simulink model "WormAndGearConstraint0x5B10x5D"  (R2024a)
settings: Solver=ode45  StartTime=0.0  StopTime=20  MaxStep=0.01  RelTol=1e-3
PreLoadFcn:
  | addpath(fullfile('WormAndGearConstraintSupport','Data'));
  | addpath(fullfile('WormAndGearConstraintSupport','Scripts'));
model workspace: external: MATLAB File WormAndGearConstraintParameters.m (data not in the file)
undefined symbols (not defined in the file): driveconn, frame, framemount, slewdrive, solarpanel, support, X, Y, Z
libraries: sm_lib x393, nesl_utility x10, fl_lib x4, SignalEditorBlockLib x2, fl_ps_legacy_lib x1
(part 2 of 11)

== system WormAndGearConstraint0x5B10x5D/Solar Array/Solar Tracker1/Slew Drive ==
  Housing : Subsystem
      mask Display:
      | image(fullfile('WormAndGearConstraintSupport','Images','SlewDriveHousing.png'));
      | port_label('lconn',1,'S');
      | port_label('rconn',1,'B');
  Housing xForm : sm_lib/Frames and Transforms/Rigid Transform  RotationMethod=AlignedAxes  FollAlignAxisA=+X  BaseAlignAxisA=-Y  FollAlignAxisB=+Z  BaseAlignAxisB=+Z  RotationStandardAxis=+Z  RotationAngle=0.0  RotationAngleUnits=deg  RotationArbitraryAxis=[0 0 1]  RotationSequenceAxes=FollowerAxes  RotationSequence=XYX  RotationSequenceAngles=[0 0 0]  RotationSequenceAnglesUnits=deg  RotationMatrix=[1 0 0; 0 1 0; 0 0 1]  Quaternion=[1 0 0 0]  TranslationMethod=StandardAxis  TranslationCartesianOffset=[0 0 0]  TranslationCartesianOffsetUnits=m  TranslationStandardAxis=+Y  TranslationStandardOffset=housingOffset  TranslationStandardOffsetUnits=m  TranslationROffset=0  TranslationROffsetUnits=m  TranslationThetaOffset=0  TranslationThetaOffsetUnits=deg  TranslationZOffset=0  TranslationZOffsetUnits=m
  Root Frame : sm_lib/Frames and Transforms/Reference Frame
  Worm and Gear Assembly : Subsystem
      mask Display:
      | image(fullfile('WormAndGearConstraintSupport','Images','SlewDriveWormAndGear.png'));
      | port_label('lconn',1,'R');
      | port_label('lconn',2,'qGear');
      | port_label('rconn',1,'T');
      | port_label('rconn',2,'wWorm');
      | port_label('rconn',3,'tWorm');
  B : PMIOPort  Side=Left
  T : PMIOPort  Port=2  Side=Right
  qGear : PMIOPort  Port=3  Side=Left
  wWorm : PMIOPort  Port=4  Side=Right
  tWorm : PMIOPort  Port=5  Side=Right
  connections:
  qGear/RConn1 -- Worm and Gear Assembly/LConn2
  tWorm/RConn1 -- Worm and Gear Assembly/RConn3
  Worm and Gear Assembly/RConn2 -- wWorm/RConn1
  T/RConn1 -- Worm and Gear Assembly/RConn1
  Housing xForm/LConn1 -- Worm and Gear Assembly/LConn1 -- Root Frame/RConn1
  B/RConn1 -- Housing/RConn1
  Housing/LConn1 -- Housing xForm/RConn1

== system WormAndGearConstraint0x5B10x5D/Solar Array/Solar Tracker1/Solar Panel Assembly ==
  Frame : Subsystem  AncestorBlock=WormAndGearConstraintLibrary/Frame  mask(Frame){width=frame.width, height=frame.height, depth=frame.depth, beamWidth=frame.beamWidth, beamThickness=frame.beamThickness, frameWidth=frame.frameWidth, frameThickness=frame.frameThickness, rho=frame.density, beamColor=frame.beamColor, frameColor=frame.frameColor}
      mask prompts: width "Width (m)"; height "Height (m)"; depth "Depth (m)"; beamWidth "Beam Width (m)"; beamThickness "Beam Thickness (m)"; frameWidth "Frame Width (m)"; frameThickness "Frame Thickness (m)"; rho "Density (kg/m^3)"; beamColor "Beam Color [r g b]"; frameColor "Frame Color [r g b]"
      mask help:
      | This block models the mounting frame of the solar tracker.
      |
      | Port B corresponds to the center of the base face of the horizontal beam. Port T corresponds to the center of the top face of the horizontal beam.
      mask init:
      | horizBeamLength = width - 2*frameWidth;
      | vertBeamLength = height - 2*frameWidth;
      | 
      | vertBeam1_offset = [-0.5*vertBeamLength 0 -(1/3)*horizBeamLength];
      | vertBeam2_offset = [-0.5*vertBeamLength 0 -(2/3)*horizBeamLength];
      | 
      | baseOffset = [0 -0.5*depth 0.5*horizBeamLength];
      | topOffset  = [0  0.5*depth 0.5*horizBeamLength];
      | 
      | leftFrameOffset  = [-0.5*height 0 -0.5*frameWidth];
      | rightFrameOffset = [-0.5*height 0  0.5*frameWidth];
      | 
      | nearFarFrameOffset = 0.5*height-0.5*frameWidth;
      settings: LibrarySourceBlock=sm_solar_tracker_lib/Frame
      mask DialogControl Tab1 Prompt: Dimensions
      mask DialogControl Tab2 Prompt: Material Properties
      mask Display:
      | image(fullfile('WormAndGearConstraintSupport','Images','Frame.png'));
      | port_label('lconn',1,'B');
      | port_label('rconn',1,'T');
  Frame Mount : Subsystem  AncestorBlock=WormAndGearConstraintLibrary/Frame Mount  mask(Frame Mount){bracketWidth=framemount.bracketWidthHeight, bracketThickness=framemount.bracketThickness, bracketOffset=framemount.bracketOffset, holeRadius=framemount.holeRadius, holeOffset=framemount.holeOffset, baseThickness=framemount.baseThickness, rho=framemount.density, mountColor=framemount.mountColor, pinColor=framemount.pinColor}
      mask prompts: bracketWidth "Bracket Width and Height (m)"; bracketThickness "Bracket Thickness (m)"; bracketOffset "Bracket Offset (m)"; holeRadius "Hole Radius (m)"; holeOffset "Hole Offset (m)"; baseThickness "Base Thickness (m)"; rho "Density (kg/m^3)"; mountColor "Mount Color [r g b]"; pinColor "Pin Color [r g b]"
      mask help:
      | This block models the mount for the frame of the solar tracker.
      |
      | Port B corresponds to the center of the base plate. Port H corresponds to the center point of the pin that passes through the holes of the bracket.
      mask init:
      | baseAngle = atan(bracketWidth / (bracketOffset + bracketThickness));
      | baseRadius = 0.5*bracketWidth / sin(baseAngle);
      | pinLength = bracketOffset + bracketThickness;
      settings: LibrarySourceBlock=sm_solar_tracker_lib/Frame Mount
      mask DialogControl Tab1 Prompt: Dimensions
      mask DialogControl Tab2 Prompt: Material Properties
      mask Display:
      | image(fullfile('WormAndGearConstraintSupport','Images','FrameMount.png'));
      | port_label('lconn',1,'B');
      | port_label('rconn',1,'H');
  Solar Panel : Subsystem  AncestorBlock=WormAndGearConstraintLibrary/Solar Panel  mask(Solar Panel){width=solarpanel.width, height=solarpanel.height, frameWidth=solarpanel.frameWidth, frameDepth=solarpanel.frameDepth, cellsRho=solarpanel.cellDensity, frameRho=solarpanel.frameDensity, cellsColor=solarpanel.cellColor, frameColor=solarpanel.frameColor}
      mask prompts: width "Width (m)"; height "Height (m)"; frameWidth "Frame Width (m)"; frameDepth "Frame Depth (m)"; cellsRho "Cell Density (kg/m^3)"; frameRho "Frame Density (kg/m^3)"; cellsColor "Cell Color [r g b]"; frameColor "Frame Color [r g b]"
      mask help:
      | This block models the solar panel of the solar tracker.
      |
      | Port B corresponds to the center of the base face.
      mask init:
      | % Solar cells
      | cellsDim = ...
      |   [width-2*frameWidth, height-2*frameWidth, 0.25*frameDepth];
      | 
      | % Frame base and edges
      | frameBaseDim = [width height 0.25*frameDepth];
      | frameVertEdgeDim = [frameWidth height 0.75*frameDepth];
      | frameHorizEdgeDim = [width-2*frameWidth frameWidth 0.75*frameDepth];
      | 
      | % Horizontal dividers
      | frameMajorHorizDim = frameHorizEdgeDim;
      | frameMinorHorizDim = ...
      |   [width-2*frameWidth 0.5*frameWidth 0.25*frameDepth];
      | 
      | frameMinorHorizSpacing = (1/12)*(height-frameWidth);
      | frameMinorHorizOffsetZ = -0.25*frameDepth;
      | 
      | frameMinorHoriz1_offset  = ...
      |   [0  5*frameMinorHorizSpacing frameMinorHorizOffsetZ];
      | frameMinorHoriz2_offset  = ...
      |   [0  4*frameMinorHorizSpacing frameMinorHorizOffsetZ];
      | frameMinorHoriz3_offset  = ...
      |   [0  3*frameMinorHorizSpacing frameMinorHorizOffsetZ];
      | frameMinorHoriz4_offset  = ...
      |   [0  2*frameMinorHorizSpacing frameMinorHorizOffsetZ];
      | frameMinorHoriz5_offset  = ...
      |   [0  1*frameMinorHorizSpacing frameMinorHorizOffsetZ];
      | frameMinorHoriz6_offset  = ...
      |   [0 -1*frameMinorHorizSpacing frameMinorHorizOffsetZ];
      | frameMinorHoriz7_offset  = ...
      |   [0 -2*frameMinorHorizSpacing frameMinorHorizOffsetZ];
      | frameMinorHoriz8_offset  = ...
      |   [0 -3*frameMinorHorizSpacing frameMinorHorizOffsetZ];
      | frameMinorHoriz9_offset  = ...
      |   [0 -4*frameMinorHorizSpacing frameMinorHorizOffsetZ];
      | frameMinorHoriz10_offset = ...
      |   [0 -5*frameMinorHorizSpacing frameMinorHorizOffsetZ];
      | 
      | % Vertical dividers
      | frameMajorVertDim = ...
      |   [frameWidth height-2*frameWidth 0.5*frameDepth];
      | frameMinorVertDim = ...
      |   [0.25*frameWidth height-2*frameWidth 0.125*frameDepth];
      | 
      | frameMajorVertOffset = (1/6)*width;
      | frameMinorVertSpacing = (1/18)*(width-frameWidth);
      | frameMinorVertOffsetZ = -(0.5*frameDepth-frameMinorVertDim(3));
      | 
      | frameMinorVert1_offset = ...
      |   [-7*frameMinorVertSpacing 0 frameMinorVertOffsetZ];
      | frameMinorVert2_offset = ...
      |   [-5*frameMinorVertSpacing 0 frameMinorVertOffsetZ];
      | frameMinorVert3_offset = ...
      |   [-1*frameMinorVertSpacing 0 frameMinorVertOffsetZ];
      | frameMinorVert4_offset = ...
      |   [ 1*frameMinorVertSpacing 0 frameMinorVertOffsetZ];
      | frameMinorVert5_offset = ...
      |   [ 5*frameMinorVertSpacing 0 frameMinorVertOffsetZ];
      | frameMinorVert6_offset = ...
      |   [ 7*frameMinorVertSpacing 0 frameMinorVertOffsetZ];
      settings: LibrarySourceBlock=sm_solar_tracker_lib/Solar Panel
      mask DialogControl Tab1 Prompt: Dimensions
      mask DialogControl Tab2 Prompt: Material Properties
      mask Display:
      | image(fullfile('WormAndGearConstraintSupport','Images','SolarPanel.png'));
      | port_label('lconn',1,'B');
  H : PMIOPort  Side=Left
  connections:
  Frame/RConn1 -- Solar Panel/LConn1
  Frame Mount/LConn1 -- Frame/LConn1
  H/RConn1 -- Frame Mount/RConn1

== system WormAndGearConstraint0x5B10x5D/Solar Array/Solar Tracker1/Support ==
  Base : sm_lib/Body Elements/Extruded Solid  ExtrusionType=General  PolygonNumSides=3  PolygonOuterRadius=1  PolygonOuterRadiusUnits=m  ExportEntireGeometry=off  ExtrusionCrossSection=baseVertices  ExtrusionCrossSectionUnits=m  ExportConvexHullGeometry=off  ExtrusionLength=baseThickness  ExtrusionLengthUnits=m  InertiaType=CalculateFromGeometry  BasedOnType=Density  Density=rho  DensityUnits=kg/m^3  Mass=1  MassUnits=kg  CenterOfMass=[0 0 0]  CenterOfMassUnits=m  MomentsOfInertia=[1 1 1]  MomentsOfInertiaUnits=kg*m^2  ProductsOfInertia=[1 1 1]  ProductsOfInertiaUnits=kg*m^2  GraphicType=FromGeometry  MarkerShape=Sphere  MarkerSize=10  GraphicVisPropType=SimpleVisualProperties  GraphicDiffuseColor=color  GraphicOpacity=1.0  GraphicSpecularColor=[0.5 0.5 0.5 1.0]  GraphicAmbientColor=[0.15 0.15 0.15 1.0]  GraphicEmissiveColor=[0.0 0.0 0.0 1.0]  GraphicShininess=75  DoExposeReferenceFrame=off  SerializedFrames=<Frames><Frame><Id>Frame1</Id><Value><Name>B</Name><Origin><Source>GeometricFeature</Source><FeatureName>bottom surface</FeatureName></Origin><PrimaryAxis><DefinedDirection>+Z</DefinedDirection><Source>ReferenceFrame</Source><SourceDirection>+Z</SourceDirection><FeatureName></FeatureName></PrimaryAxis><SecondaryAxis><DefinedDirection>+X</DefinedDirection><Source>ReferenceFrame</Source><SourceDirection>+X</SourceDirection><FeatureName></FeatureName></SecondaryAxis></Value></Frame><Frame><Id>Frame2</Id><Value><Name>T</Name><Origin><Source>GeometricFeature</Source><FeatureName>top surface</FeatureName></Origin><PrimaryAxis><DefinedDirection>+Z</DefinedDirection><Source>ReferenceFrame</Source><SourceDirection>+Z</SourceDirection><FeatureName></FeatureName></PrimaryAxis><SecondaryAxis><DefinedDirection>+X</DefinedDirection><Source>ReferenceFrame</Source><SourceDirection>+X</SourceDirection><FeatureName></FeatureName></SecondaryAxis></Value></Frame></Frames>
  Column : Subsystem  AncestorBlock=WormAndGearConstraintLibrary/Hollow Cylinder  mask(Hollow Cylinder){outerRadius=columnRadius, thickness=columnThickness, length=columnHeight, rho=rho, color=color}
      mask prompts: outerRadius "Outer Radius (m)"; thickness "Thickness (m)"; length "Length (m)"; rho "Density (kg/m^3)"; color "Color [r g b]"
      mask help:
      | This block models a hollow cylinder element.
      |
      | Port L corresponds to the left-hand end of the cylinder. Port R corresponds to the right-hand end of the cylinder.
      mask init: same as WormAndGearConstraint0x5B10x5D/Solar Array/Solar Tracker1/Drive Connection/Drive Connection
      mask DialogControl Tab1 Prompt: Dimensions
      mask DialogControl Tab2 Prompt: Material Properties
      mask Display:
      | image(fullfile('WormAndGearConstraintSupport','Images','HollowCylinder.png'));
      | port_label('lconn',1,'L');
      | port_label('rconn',1,'R');
  B : PMIOPort  Side=Left
  T : PMIOPort  Port=2  Side=Right
  connections:
  Column/RConn1 -- T/RConn1
  Column/LConn1 -- Base/RConn1
  Base/LConn1 -- B/RConn1

== system WormAndGearConstraint0x5B10x5D/Solar Array/Solar Tracker2/Drive Connection ==
  Bracket : Subsystem  AncestorBlock=WormAndGearConstraintLibrary/Single Bracket  mask(Single Bracket){height=bracketWidth, width=bracketWidth, thickness=bracketThickness, holeOffset=holeOffset, holeRadius=holeRadius, rho=rho, color=color}
      mask prompts: height "Height (m)"; width "Width (m)"; thickness "Thickness (m)"; holeOffset "Hole Offset (m)"; holeRadius "Hole Radius (m)"; rho "Density (kg/m^3)"; color "Color [r g b]"
      mask help:
      | This block models a bracket element.
      |
      | Port B corresponds to the center point of the base face. Port H corresponds to the center of the hole.
      mask DialogControl Tab1 Prompt: Dimensions
      mask DialogControl Tab2 Prompt: Material Properties
      mask Display:
      | image(fullfile('WormAndGearConstraintSupport','Images','SingleBracket.png'));
      | port_label('lconn',1,'B');
      | port_label('rconn',1,'H');
  Bracket Base : sm_lib/Body Elements/Cylindrical Solid  CylinderRadius=baseRadius  CylinderRadiusUnits=m  CylinderLength=baseThickness  CylinderLengthUnits=m  ExportEntireGeometry=off  InertiaType=CalculateFromGeometry  BasedOnType=Density  Density=rho  DensityUnits=kg/m^3  Mass=1  MassUnits=kg  CenterOfMass=[0 0 0]  CenterOfMassUnits=m  MomentsOfInertia=[1 1 1]  MomentsOfInertiaUnits=kg*m^2  ProductsOfInertia=[1 1 1]  ProductsOfInertiaUnits=kg*m^2  GraphicType=FromGeometry  MarkerShape=Sphere  MarkerSize=10  GraphicVisPropType=SimpleVisualProperties  GraphicDiffuseColor=color  GraphicOpacity=1.0  GraphicSpecularColor=[0.5 0.5 0.5 1.0]  GraphicAmbientColor=[0.15 0.15 0.15 1.0]  GraphicEmissiveColor=[0.0 0.0 0.0 1.0]  GraphicShininess=75  DoExposeReferenceFrame=off  SerializedFrames=<Frames><Frame><Id>Frame1</Id><Value><Name>T</Name><Origin><Source>GeometricFeature</Source><FeatureName>top surface</FeatureName></Origin><PrimaryAxis><DefinedDirection>+Z</DefinedDirection><Source>ReferenceFrame</Source><SourceDirection>+Z</SourceDirection><FeatureName></FeatureName></PrimaryAxis><SecondaryAxis><DefinedDirection>+X</DefinedDirection><Source>ReferenceFrame</Source><SourceDirection>-Y</SourceDirection><FeatureName></FeatureName></SecondaryAxis></Value></Frame><Frame><Id>Frame2</Id><Value><Name>B</Name><Origin><Source>GeometricFeature</Source><FeatureName>bottom surface</FeatureName></Origin><PrimaryAxis><DefinedDirection>+Z</DefinedDirection><Source>ReferenceFrame</Source><SourceDirection>+Z</SourceDirection><FeatureName></FeatureName></PrimaryAxis><SecondaryAxis><DefinedDirection>+X</DefinedDirection><Source>ReferenceFrame</Source><SourceDirection>+X</SourceDirection><FeatureName></FeatureName></SecondaryAxis></Value></Frame></Frames>
  Drive Connection : Subsystem  AncestorBlock=WormAndGearConstraintLibrary/Hollow Cylinder  mask(Hollow Cylinder){outerRadius=connRadius, thickness=connThickness, length=connLength, rho=rho, color=color}
      mask prompts: outerRadius "Outer Radius (m)"; thickness "Thickness (m)"; length "Length (m)"; rho "Density (kg/m^3)"; color "Color [r g b]"
      mask help:
      | This block models a hollow cylinder element.
      |
      | Port L corresponds to the left-hand end of the cylinder. Port R corresponds to the right-hand end of the cylinder.
      mask init: same as WormAndGearConstraint0x5B10x5D/Solar Array/Solar Tracker1/Drive Connection/Drive Connection
      mask DialogControl Tab1 Prompt: Dimensions
      mask DialogControl Tab2 Prompt: Material Properties
      mask Display:
      | image(fullfile('WormAndGearConstraintSupport','Images','HollowCylinder.png'));
      | port_label('lconn',1,'L');
      | port_label('rconn',1,'R');
  B : PMIOPort  Side=Left
  H : PMIOPort  Port=2  Side=Right
  connections:
  Drive Connection/LConn1 -- B/RConn1
  Drive Connection/RConn1 -- Bracket Base/RConn1
  Bracket Base/LConn1 -- Bracket/LConn1
  H/RConn1 -- Bracket/RConn1

== system WormAndGearConstraint0x5B10x5D/Solar Array/Solar Tracker2/Slew Drive ==
  Housing : Subsystem
      mask Display:
      | image(fullfile('WormAndGearConstraintSupport','Images','SlewDriveHousing.png'));
      | port_label('lconn',1,'S');
      | port_label('rconn',1,'B');
  Housing xForm : sm_lib/Frames and Transforms/Rigid Transform  RotationMethod=AlignedAxes  FollAlignAxisA=+X  BaseAlignAxisA=-Y  FollAlignAxisB=+Z  BaseAlignAxisB=+Z  RotationStandardAxis=+Z  RotationAngle=0.0  RotationAngleUnits=deg  RotationArbitraryAxis=[0 0 1]  RotationSequenceAxes=FollowerAxes  RotationSequence=XYX  RotationSequenceAngles=[0 0 0]  RotationSequenceAnglesUnits=deg  RotationMatrix=[1 0 0; 0 1 0; 0 0 1]  Quaternion=[1 0 0 0]  TranslationMethod=StandardAxis  TranslationCartesianOffset=[0 0 0]  TranslationCartesianOffsetUnits=m  TranslationStandardAxis=+Y  TranslationStandardOffset=housingOffset  TranslationStandardOffsetUnits=m  TranslationROffset=0  TranslationROffsetUnits=m  TranslationThetaOffset=0  TranslationThetaOffsetUnits=deg  TranslationZOffset=0  TranslationZOffsetUnits=m
  Root Frame : sm_lib/Frames and Transforms/Reference Frame
  Worm and Gear Assembly : Subsystem
      mask Display:
      | image(fullfile('WormAndGearConstraintSupport','Images','SlewDriveWormAndGear.png'));
      | port_label('lconn',1,'R');
      | port_label('lconn',2,'qGear');
      | port_label('rconn',1,'T');
      | port_label('rconn',2,'wWorm');
      | port_label('rconn',3,'tWorm');
  B : PMIOPort  Side=Left
  T : PMIOPort  Port=2  Side=Right
  qGear : PMIOPort  Port=3  Side=Left
  wWorm : PMIOPort  Port=4  Side=Right
  tWorm : PMIOPort  Port=5  Side=Right
  connections:
  qGear/RConn1 -- Worm and Gear Assembly/LConn2
  tWorm/RConn1 -- Worm and Gear Assembly/RConn3
  Worm and Gear Assembly/RConn2 -- wWorm/RConn1
  T/RConn1 -- Worm and Gear Assembly/RConn1
  Housing xForm/LConn1 -- Worm and Gear Assembly/LConn1 -- Root Frame/RConn1
  B/RConn1 -- Housing/RConn1
  Housing/LConn1 -- Housing xForm/RConn1

== system WormAndGearConstraint0x5B10x5D/Solar Array/Solar Tracker2/Solar Panel Assembly ==
  Frame : Subsystem  AncestorBlock=WormAndGearConstraintLibrary/Frame  mask(Frame){width=frame.width, height=frame.height, depth=frame.depth, beamWidth=frame.beamWidth, beamThickness=frame.beamThickness, frameWidth=frame.frameWidth, frameThickness=frame.frameThickness, rho=frame.density, beamColor=frame.beamColor, frameColor=frame.frameColor}
      mask prompts: width "Width (m)"; height "Height (m)"; depth "Depth (m)"; beamWidth "Beam Width (m)"; beamThickness "Beam Thickness (m)"; frameWidth "Frame Width (m)"; frameThickness "Frame Thickness (m)"; rho "Density (kg/m^3)"; beamColor "Beam Color [r g b]"; frameColor "Frame Color [r g b]"
      mask help:
      | This block models the mounting frame of the solar tracker.
      |
      | Port B corresponds to the center of the base face of the horizontal beam. Port T corresponds to the center of the top face of the horizontal beam.
      mask init: same as WormAndGearConstraint0x5B10x5D/Solar Array/Solar Tracker1/Solar Panel Assembly/Frame
      settings: LibrarySourceBlock=sm_solar_tracker_lib/Frame
      mask DialogControl Tab1 Prompt: Dimensions
      mask DialogControl Tab2 Prompt: Material Properties
      mask Display:
      | image(fullfile('WormAndGearConstraintSupport','Images','Frame.png'));
      | port_label('lconn',1,'B');
      | port_label('rconn',1,'T');
  Frame Mount : Subsystem  AncestorBlock=WormAndGearConstraintLibrary/Frame Mount  mask(Frame Mount){bracketWidth=framemount.bracketWidthHeight, bracketThickness=framemount.bracketThickness, bracketOffset=framemount.bracketOffset, holeRadius=framemount.holeRadius, holeOffset=framemount.holeOffset, baseThickness=framemount.baseThickness, rho=framemount.density, mountColor=framemount.mountColor, pinColor=framemount.pinColor}
      mask prompts: bracketWidth "Bracket Width and Height (m)"; bracketThickness "Bracket Thickness (m)"; bracketOffset "Bracket Offset (m)"; holeRadius "Hole Radius (m)"; holeOffset "Hole Offset (m)"; baseThickness "Base Thickness (m)"; rho "Density (kg/m^3)"; mountColor "Mount Color [r g b]"; pinColor "Pin Color [r g b]"
      mask help:
      | This block models the mount for the frame of the solar tracker.
      |
      | Port B corresponds to the center of the base plate. Port H corresponds to the center point of the pin that passes through the holes of the bracket.
      mask init:
      | baseAngle = atan(bracketWidth / (bracketOffset + bracketThickness));
      | baseRadius = 0.5*bracketWidth / sin(baseAngle);
      | pinLength = bracketOffset + bracketThickness;
      settings: LibrarySourceBlock=sm_solar_tracker_lib/Frame Mount
      mask DialogControl Tab1 Prompt: Dimensions
      mask DialogControl Tab2 Prompt: Material Properties
      mask Display:
      | image(fullfile('WormAndGearConstraintSupport','Images','FrameMount.png'));
      | port_label('lconn',1,'B');
      | port_label('rconn',1,'H');
  Solar Panel : Subsystem  AncestorBlock=WormAndGearConstraintLibrary/Solar Panel  mask(Solar Panel){width=solarpanel.width, height=solarpanel.height, frameWidth=solarpanel.frameWidth, frameDepth=solarpanel.frameDepth, cellsRho=solarpanel.cellDensity, frameRho=solarpanel.frameDensity, cellsColor=solarpanel.cellColor, frameColor=solarpanel.frameColor}
      mask prompts: width "Width (m)"; height "Height (m)"; frameWidth "Frame Width (m)"; frameDepth "Frame Depth (m)"; cellsRho "Cell Density (kg/m^3)"; frameRho "Frame Density (kg/m^3)"; cellsColor "Cell Color [r g b]"; frameColor "Frame Color [r g b]"
      mask help:
      | This block models the solar panel of the solar tracker.
      |
      | Port B corresponds to the center of the base face.
      mask init: same as WormAndGearConstraint0x5B10x5D/Solar Array/Solar Tracker1/Solar Panel Assembly/Solar Panel
      settings: LibrarySourceBlock=sm_solar_tracker_lib/Solar Panel
      mask DialogControl Tab1 Prompt: Dimensions
      mask DialogControl Tab2 Prompt: Material Properties
      mask Display:
      | image(fullfile('WormAndGearConstraintSupport','Images','SolarPanel.png'));
      | port_label('lconn',1,'B');
  H : PMIOPort  Side=Left
  connections:
  H/RConn1 -- Frame Mount/RConn1
  Frame Mount/LConn1 -- Frame/LConn1
  Frame/RConn1 -- Solar Panel/LConn1

== system WormAndGearConstraint0x5B10x5D/Solar Array/Solar Tracker2/Support ==
  Base : sm_lib/Body Elements/Extruded Solid  ExtrusionType=General  PolygonNumSides=3  PolygonOuterRadius=1  PolygonOuterRadiusUnits=m  ExportEntireGeometry=off  ExtrusionCrossSection=baseVertices  ExtrusionCrossSectionUnits=m  ExportConvexHullGeometry=off  ExtrusionLength=baseThickness  ExtrusionLengthUnits=m  InertiaType=CalculateFromGeometry  BasedOnType=Density  Density=rho  DensityUnits=kg/m^3  Mass=1  MassUnits=kg  CenterOfMass=[0 0 0]  CenterOfMassUnits=m  MomentsOfInertia=[1 1 1]  MomentsOfInertiaUnits=kg*m^2  ProductsOfInertia=[1 1 1]  ProductsOfInertiaUnits=kg*m^2  GraphicType=FromGeometry  MarkerShape=Sphere  MarkerSize=10  GraphicVisPropType=SimpleVisualProperties  GraphicDiffuseColor=color  GraphicOpacity=1.0  GraphicSpecularColor=[0.5 0.5 0.5 1.0]  GraphicAmbientColor=[0.15 0.15 0.15 1.0]  GraphicEmissiveColor=[0.0 0.0 0.0 1.0]  GraphicShininess=75  DoExposeReferenceFrame=off  SerializedFrames=<Frames><Frame><Id>Frame1</Id><Value><Name>B</Name><Origin><Source>GeometricFeature</Source><FeatureName>bottom surface</FeatureName></Origin><PrimaryAxis><DefinedDirection>+Z</DefinedDirection><Source>ReferenceFrame</Source><SourceDirection>+Z</SourceDirection><FeatureName></FeatureName></PrimaryAxis><SecondaryAxis><DefinedDirection>+X</DefinedDirection><Source>ReferenceFrame</Source><SourceDirection>+X</SourceDirection><FeatureName></FeatureName></SecondaryAxis></Value></Frame><Frame><Id>Frame2</Id><Value><Name>T</Name><Origin><Source>GeometricFeature</Source><FeatureName>top surface</FeatureName></Origin><PrimaryAxis><DefinedDirection>+Z</DefinedDirection><Source>ReferenceFrame</Source><SourceDirection>+Z</SourceDirection><FeatureName></FeatureName></PrimaryAxis><SecondaryAxis><DefinedDirection>+X</DefinedDirection><Source>ReferenceFrame</Source><SourceDirection>+X</SourceDirection><FeatureName></FeatureName></SecondaryAxis></Value></Frame></Frames>
  Column : Subsystem  AncestorBlock=WormAndGearConstraintLibrary/Hollow Cylinder  mask(Hollow Cylinder){outerRadius=columnRadius, thickness=columnThickness, length=columnHeight, rho=rho, color=color}
      mask prompts: outerRadius "Outer Radius (m)"; thickness "Thickness (m)"; length "Length (m)"; rho "Density (kg/m^3)"; color "Color [r g b]"
      mask help:
      | This block models a hollow cylinder element.
      |
      | Port L corresponds to the left-hand end of the cylinder. Port R corresponds to the right-hand end of the cylinder.
      mask init: same as WormAndGearConstraint0x5B10x5D/Solar Array/Solar Tracker1/Drive Connection/Drive Connection
      mask DialogControl Tab1 Prompt: Dimensions
      mask DialogControl Tab2 Prompt: Material Properties
      mask Display:
      | image(fullfile('WormAndGearConstraintSupport','Images','HollowCylinder.png'));
      | port_label('lconn',1,'L');
      | port_label('rconn',1,'R');
  B : PMIOPort  Side=Left
  T : PMIOPort  Port=2  Side=Right
  connections:
  Column/RConn1 -- T/RConn1
  Column/LConn1 -- Base/RConn1
  Base/LConn1 -- B/RConn1

== system WormAndGearConstraint0x5B10x5D/Solar Array/Solar Tracker3/Drive Connection ==
  Bracket : Subsystem  AncestorBlock=WormAndGearConstraintLibrary/Single Bracket  mask(Single Bracket){height=bracketWidth, width=bracketWidth, thickness=bracketThickness, holeOffset=holeOffset, holeRadius=holeRadius, rho=rho, color=color}
      mask prompts: height "Height (m)"; width "Width (m)"; thickness "Thickness (m)"; holeOffset "Hole Offset (m)"; holeRadius "Hole Radius (m)"; rho "Density (kg/m^3)"; color "Color [r g b]"
      mask help:
      | This block models a bracket element.
      |
      | Port B corresponds to the center point of the base face. Port H corresponds to the center of the hole.
      mask DialogControl Tab1 Prompt: Dimensions
      mask DialogControl Tab2 Prompt: Material Properties
      mask Display:
      | image(fullfile('WormAndGearConstraintSupport','Images','SingleBracket.png'));
      | port_label('lconn',1,'B');
      | port_label('rconn',1,'H');
  Bracket Base : sm_lib/Body Elements/Cylindrical Solid  CylinderRadius=baseRadius  CylinderRadiusUnits=m  CylinderLength=baseThickness  CylinderLengthUnits=m  ExportEntireGeometry=off  InertiaType=CalculateFromGeometry  BasedOnType=Density  Density=rho  DensityUnits=kg/m^3  Mass=1  MassUnits=kg  CenterOfMass=[0 0 0]  CenterOfMassUnits=m  MomentsOfInertia=[1 1 1]  MomentsOfInertiaUnits=kg*m^2  ProductsOfInertia=[1 1 1]  ProductsOfInertiaUnits=kg*m^2  GraphicType=FromGeometry  MarkerShape=Sphere  MarkerSize=10  GraphicVisPropType=SimpleVisualProperties  GraphicDiffuseColor=color  GraphicOpacity=1.0  GraphicSpecularColor=[0.5 0.5 0.5 1.0]  GraphicAmbientColor=[0.15 0.15 0.15 1.0]  GraphicEmissiveColor=[0.0 0.0 0.0 1.0]  GraphicShininess=75  DoExposeReferenceFrame=off  SerializedFrames=<Frames><Frame><Id>Frame1</Id><Value><Name>T</Name><Origin><Source>GeometricFeature</Source><FeatureName>top surface</FeatureName></Origin><PrimaryAxis><DefinedDirection>+Z</DefinedDirection><Source>ReferenceFrame</Source><SourceDirection>+Z</SourceDirection><FeatureName></FeatureName></PrimaryAxis><SecondaryAxis><DefinedDirection>+X</DefinedDirection><Source>ReferenceFrame</Source><SourceDirection>-Y</SourceDirection><FeatureName></FeatureName></SecondaryAxis></Value></Frame><Frame><Id>Frame2</Id><Value><Name>B</Name><Origin><Source>GeometricFeature</Source><FeatureName>bottom surface</FeatureName></Origin><PrimaryAxis><DefinedDirection>+Z</DefinedDirection><Source>ReferenceFrame</Source><SourceDirection>+Z</SourceDirection><FeatureName></FeatureName></PrimaryAxis><SecondaryAxis><DefinedDirection>+X</DefinedDirection><Source>ReferenceFrame</Source><SourceDirection>+X</SourceDirection><FeatureName></FeatureName></SecondaryAxis></Value></Frame></Frames>
  Drive Connection : Subsystem  AncestorBlock=WormAndGearConstraintLibrary/Hollow Cylinder  mask(Hollow Cylinder){outerRadius=connRadius, thickness=connThickness, length=connLength, rho=rho, color=color}
      mask prompts: outerRadius "Outer Radius (m)"; thickness "Thickness (m)"; length "Length (m)"; rho "Density (kg/m^3)"; color "Color [r g b]"
      mask help:
      | This block models a hollow cylinder element.
      |
      | Port L corresponds to the left-hand end of the cylinder. Port R corresponds to the right-hand end of the cylinder.
      mask init: same as WormAndGearConstraint0x5B10x5D/Solar Array/Solar Tracker1/Drive Connection/Drive Connection
      mask DialogControl Tab1 Prompt: Dimensions
      mask DialogControl Tab2 Prompt: Material Properties
      mask Display:
      | image(fullfile('WormAndGearConstraintSupport','Images','HollowCylinder.png'));
      | port_label('lconn',1,'L');
      | port_label('rconn',1,'R');
  B : PMIOPort  Side=Left
  H : PMIOPort  Port=2  Side=Right
  connections:
  Drive Connection/LConn1 -- B/RConn1
  Drive Connection/RConn1 -- Bracket Base/RConn1
  Bracket Base/LConn1 -- Bracket/LConn1
  H/RConn1 -- Bracket/RConn1

== system WormAndGearConstraint0x5B10x5D/Solar Array/Solar Tracker3/Slew Drive ==
  Housing : Subsystem
      mask Display:
      | image(fullfile('WormAndGearConstraintSupport','Images','SlewDriveHousing.png'));
      | port_label('lconn',1,'S');
      | port_label('rconn',1,'B');
  Housing xForm : sm_lib/Frames and Transforms/Rigid Transform  RotationMethod=AlignedAxes  FollAlignAxisA=+X  BaseAlignAxisA=-Y  FollAlignAxisB=+Z  BaseAlignAxisB=+Z  RotationStandardAxis=+Z  RotationAngle=0.0  RotationAngleUnits=deg  RotationArbitraryAxis=[0 0 1]  RotationSequenceAxes=FollowerAxes  RotationSequence=XYX  RotationSequenceAngles=[0 0 0]  RotationSequenceAnglesUnits=deg  RotationMatrix=[1 0 0; 0 1 0; 0 0 1]  Quaternion=[1 0 0 0]  TranslationMethod=StandardAxis  TranslationCartesianOffset=[0 0 0]  TranslationCartesianOffsetUnits=m  TranslationStandardAxis=+Y  TranslationStandardOffset=housingOffset  TranslationStandardOffsetUnits=m  TranslationROffset=0  TranslationROffsetUnits=m  TranslationThetaOffset=0  TranslationThetaOffsetUnits=deg  TranslationZOffset=0  TranslationZOffsetUnits=m
  Root Frame : sm_lib/Frames and Transforms/Reference Frame
  Worm and Gear Assembly : Subsystem
      mask Display:
      | image(fullfile('WormAndGearConstraintSupport','Images','SlewDriveWormAndGear.png'));
      | port_label('lconn',1,'R');
      | port_label('lconn',2,'qGear');
      | port_label('rconn',1,'T');
      | port_label('rconn',2,'wWorm');
      | port_label('rconn',3,'tWorm');
  B : PMIOPort  Side=Left
  T : PMIOPort  Port=2  Side=Right
  qGear : PMIOPort  Port=3  Side=Left
  wWorm : PMIOPort  Port=4  Side=Right
  tWorm : PMIOPort  Port=5  Side=Right
  connections:
  qGear/RConn1 -- Worm and Gear Assembly/LConn2
  tWorm/RConn1 -- Worm and Gear Assembly/RConn3
  Worm and Gear Assembly/RConn2 -- wWorm/RConn1
  T/RConn1 -- Worm and Gear Assembly/RConn1
  Housing xForm/LConn1 -- Worm and Gear Assembly/LConn1 -- Root Frame/RConn1
  B/RConn1 -- Housing/RConn1
  Housing/LConn1 -- Housing xForm/RConn1

== system WormAndGearConstraint0x5B10x5D/Solar Array/Solar Tracker3/Solar Panel Assembly ==
  Frame : Subsystem  AncestorBlock=WormAndGearConstraintLibrary/Frame  mask(Frame){width=frame.width, height=frame.height, depth=frame.depth, beamWidth=frame.beamWidth, beamThickness=frame.beamThickness, frameWidth=frame.frameWidth, frameThickness=frame.frameThickness, rho=frame.density, beamColor=frame.beamColor, frameColor=frame.frameColor}
      mask prompts: width "Width (m)"; height "Height (m)"; depth "Depth (m)"; beamWidth "Beam Width (m)"; beamThickness "Beam Thickness (m)"; frameWidth "Frame Width (m)"; frameThickness "Frame Thickness (m)"; rho "Density (kg/m^3)"; beamColor "Beam Color [r g b]"; frameColor "Frame Color [r g b]"
      mask help:
      | This block models the mounting frame of the solar tracker.
      |
      | Port B corresponds to the center of the base face of the horizontal beam. Port T corresponds to the center of the top face of the horizontal beam.
      mask init: same as WormAndGearConstraint0x5B10x5D/Solar Array/Solar Tracker1/Solar Panel Assembly/Frame
      settings: LibrarySourceBlock=sm_solar_tracker_lib/Frame
      mask DialogControl Tab1 Prompt: Dimensions
      mask DialogControl Tab2 Prompt: Material Properties
      mask Display:
      | image(fullfile('WormAndGearConstraintSupport','Images','Frame.png'));
      | port_label('lconn',1,'B');
      | port_label('rconn',1,'T');
  Frame Mount : Subsystem  AncestorBlock=WormAndGearConstraintLibrary/Frame Mount  mask(Frame Mount){bracketWidth=framemount.bracketWidthHeight, bracketThickness=framemount.bracketThickness, bracketOffset=framemount.bracketOffset, holeRadius=framemount.holeRadius, holeOffset=framemount.holeOffset, baseThickness=framemount.baseThickness, rho=framemount.density, mountColor=framemount.mountColor, pinColor=framemount.pinColor}
      mask prompts: bracketWidth "Bracket Width and Height (m)"; bracketThickness "Bracket Thickness (m)"; bracketOffset "Bracket Offset (m)"; holeRadius "Hole Radius (m)"; holeOffset "Hole Offset (m)"; baseThickness "Base Thickness (m)"; rho "Density (kg/m^3)"; mountColor "Mount Color [r g b]"; pinColor "Pin Color [r g b]"
      mask help:
      | This block models the mount for the frame of the solar tracker.
      |
      | Port B corresponds to the center of the base plate. Port H corresponds to the center point of the pin that passes through the holes of the bracket.
      mask init:
      | baseAngle = atan(bracketWidth / (bracketOffset + bracketThickness));
      | baseRadius = 0.5*bracketWidth / sin(baseAngle);
      | pinLength = bracketOffset + bracketThickness;
      settings: LibrarySourceBlock=sm_solar_tracker_lib/Frame Mount
      mask DialogControl Tab1 Prompt: Dimensions
      mask DialogControl Tab2 Prompt: Material Properties
      mask Display:
      | image(fullfile('WormAndGearConstraintSupport','Images','FrameMount.png'));
      | port_label('lconn',1,'B');
      | port_label('rconn',1,'H');
  Solar Panel : Subsystem  AncestorBlock=WormAndGearConstraintLibrary/Solar Panel  mask(Solar Panel){width=solarpanel.width, height=solarpanel.height, frameWidth=solarpanel.frameWidth, frameDepth=solarpanel.frameDepth, cellsRho=solarpanel.cellDensity, frameRho=solarpanel.frameDensity, cellsColor=solarpanel.cellColor, frameColor=solarpanel.frameColor}
      mask prompts: width "Width (m)"; height "Height (m)"; frameWidth "Frame Width (m)"; frameDepth "Frame Depth (m)"; cellsRho "Cell Density (kg/m^3)"; frameRho "Frame Density (kg/m^3)"; cellsColor "Cell Color [r g b]"; frameColor "Frame Color [r g b]"
      mask help:
      | This block models the solar panel of the solar tracker.
      |
      | Port B corresponds to the center of the base face.
      mask init: same as WormAndGearConstraint0x5B10x5D/Solar Array/Solar Tracker1/Solar Panel Assembly/Solar Panel
      settings: LibrarySourceBlock=sm_solar_tracker_lib/Solar Panel
      mask DialogControl Tab1 Prompt: Dimensions
      mask DialogControl Tab2 Prompt: Material Properties
      mask Display:
      | image(fullfile('WormAndGearConstraintSupport','Images','SolarPanel.png'));
      | port_label('lconn',1,'B');
  H : PMIOPort  Side=Left
  connections:
  Frame/RConn1 -- Solar Panel/LConn1
  Frame Mount/LConn1 -- Frame/LConn1
  H/RConn1 -- Frame Mount/RConn1

== system WormAndGearConstraint0x5B10x5D/Solar Array/Solar Tracker3/Support ==
  Base : sm_lib/Body Elements/Extruded Solid  ExtrusionType=General  PolygonNumSides=3  PolygonOuterRadius=1  PolygonOuterRadiusUnits=m  ExportEntireGeometry=off  ExtrusionCrossSection=baseVertices  ExtrusionCrossSectionUnits=m  ExportConvexHullGeometry=off  ExtrusionLength=baseThickness  ExtrusionLengthUnits=m  InertiaType=CalculateFromGeometry  BasedOnType=Density  Density=rho  DensityUnits=kg/m^3  Mass=1  MassUnits=kg  CenterOfMass=[0 0 0]  CenterOfMassUnits=m  MomentsOfInertia=[1 1 1]  MomentsOfInertiaUnits=kg*m^2  ProductsOfInertia=[1 1 1]  ProductsOfInertiaUnits=kg*m^2  GraphicType=FromGeometry  MarkerShape=Sphere  MarkerSize=10  GraphicVisPropType=SimpleVisualProperties  GraphicDiffuseColor=color  GraphicOpacity=1.0  GraphicSpecularColor=[0.5 0.5 0.5 1.0]  GraphicAmbientColor=[0.15 0.15 0.15 1.0]  GraphicEmissiveColor=[0.0 0.0 0.0 1.0]  GraphicShininess=75  DoExposeReferenceFrame=off  SerializedFrames=<Frames><Frame><Id>Frame1</Id><Value><Name>B</Name><Origin><Source>GeometricFeature</Source><FeatureName>bottom surface</FeatureName></Origin><PrimaryAxis><DefinedDirection>+Z</DefinedDirection><Source>ReferenceFrame</Source><SourceDirection>+Z</SourceDirection><FeatureName></FeatureName></PrimaryAxis><SecondaryAxis><DefinedDirection>+X</DefinedDirection><Source>ReferenceFrame</Source><SourceDirection>+X</SourceDirection><FeatureName></FeatureName></SecondaryAxis></Value></Frame><Frame><Id>Frame2</Id><Value><Name>T</Name><Origin><Source>GeometricFeature</Source><FeatureName>top surface</FeatureName></Origin><PrimaryAxis><DefinedDirection>+Z</DefinedDirection><Source>ReferenceFrame</Source><SourceDirection>+Z</SourceDirection><FeatureName></FeatureName></PrimaryAxis><SecondaryAxis><DefinedDirection>+X</DefinedDirection><Source>ReferenceFrame</Source><SourceDirection>+X</SourceDirection><FeatureName></FeatureName></SecondaryAxis></Value></Frame></Frames>
  Column : Subsystem  AncestorBlock=WormAndGearConstraintLibrary/Hollow Cylinder  mask(Hollow Cylinder){outerRadius=columnRadius, thickness=columnThickness, length=columnHeight, rho=rho, color=color}
      mask prompts: outerRadius "Outer Radius (m)"; thickness "Thickness (m)"; length "Length (m)"; rho "Density (kg/m^3)"; color "Color [r g b]"
      mask help:
      | This block models a hollow cylinder element.
      |
      | Port L corresponds to the left-hand end of the cylinder. Port R corresponds to the right-hand end of the cylinder.
      mask init: same as WormAndGearConstraint0x5B10x5D/Solar Array/Solar Tracker1/Drive Connection/Drive Connection
      mask DialogControl Tab1 Prompt: Dimensions
      mask DialogControl Tab2 Prompt: Material Properties
      mask Display:
      | image(fullfile('WormAndGearConstraintSupport','Images','HollowCylinder.png'));
      | port_label('lconn',1,'L');
      | port_label('rconn',1,'R');
  B : PMIOPort  Side=Left
  T : PMIOPort  Port=2  Side=Right
  connections:
  Column/RConn1 -- T/RConn1
  Column/LConn1 -- Base/RConn1
  Base/LConn1 -- B/RConn1

== system WormAndGearConstraint0x5B10x5D/Solar Array/Solar Tracker1/Drive Connection/Bracket ==
  Base xForm : sm_lib/Frames and Transforms/Rigid Transform  RotationMethod=AlignedAxes  FollAlignAxisA=+X  BaseAlignAxisA=+X  FollAlignAxisB=+Z  BaseAlignAxisB=+Y  RotationStandardAxis=+X  RotationAngle=90  RotationAngleUnits=deg  RotationArbitraryAxis=[0 0 1]  RotationSequenceAxes=FollowerAxes  RotationSequence=XYX  RotationSequenceAngles=[0 0 0]  RotationSequenceAnglesUnits=deg  RotationMatrix=[1 0 0; 0 1 0; 0 0 1]  Quaternion=[1 0 0 0]  TranslationMethod=None  TranslationCartesianOffset=[0 0 0]  TranslationCartesianOffsetUnits=m  TranslationStandardAxis=-Y  TranslationStandardOffset=0  TranslationStandardOffsetUnits=m  TranslationROffset=0  TranslationROffsetUnits=m  TranslationThetaOffset=0  TranslationThetaOffsetUnits=deg  TranslationZOffset=0  TranslationZOffsetUnits=m
  Bracket : Subsystem  AncestorBlock=WormAndGearConstraintLibrary/Bracket  mask(Bracket){height=height, width=width, thickness=thickness, holeOffset=holeOffset, holeRadius=holeRadius, rho=rho, color=color}
      mask prompts: height "Height (m)"; width "Width (m)"; thickness "Thickness (m)"; holeOffset "Hole Offset (m)"; holeRadius "Hole Radius (m)"; rho "Density (kg/m^3)"; color "Color [r g b]"
      mask help:
      | This block models a bracket element.
      |
      | Port B corresponds to the center point of the base face.
      mask init:
      | points = 40;
      | 
      | y = height - 0.5*width;
      | 
      | outerVertices = ...
      |   [          0      0;...
      |      0.5*width      0;...
      |      0.5*width      y;...
      |      0.5*width height;...
      |     -0.5*width height;...
      |     -0.5*width      y;...
      |     -0.5*width      0;...
      |              0      0];
      | 
      | outer = simmechanics.demohelpers.round_corners(...
      |   outerVertices, [4 5], 0.5*width, points);
      | 
      | holeTheta = linspace(1.5*pi, -0.5*pi, points);
      | 
      | hole = [holeRadius*cos(holeTheta);...
      |         holeRadius*sin(holeTheta)+holeOffset]';
      | 
      | crossSection = [hole; outer];
      mask DialogControl Tab1 Prompt: Dimensions
      mask DialogControl Tab2 Prompt: Material Properties
      mask Display:
      | image(fullfile('WormAndGearConstraintSupport','Images','Bracket.png'));
      | port_label('lconn',1,'B');
  Hole xForm : sm_lib/Frames and Transforms/Rigid Transform  RotationMethod=None  FollAlignAxisA=+X  BaseAlignAxisA=+X  FollAlignAxisB=+Y  BaseAlignAxisB=+Z  RotationStandardAxis=+X  RotationAngle=90  RotationAngleUnits=deg  RotationArbitraryAxis=[0 0 1]  RotationSequenceAxes=FollowerAxes  RotationSequence=XYX  RotationSequenceAngles=[0 0 0]  RotationSequenceAnglesUnits=deg  RotationMatrix=[1 0 0; 0 1 0; 0 0 1]  Quaternion=[1 0 0 0]  TranslationMethod=StandardAxis  TranslationCartesianOffset=[0 0 0]  TranslationCartesianOffsetUnits=m  TranslationStandardAxis=+Y  TranslationStandardOffset=holeOffset  TranslationStandardOffsetUnits=m  TranslationROffset=0  TranslationROffsetUnits=m  TranslationThetaOffset=0  TranslationThetaOffsetUnits=deg  TranslationZOffset=0  TranslationZOffsetUnits=m
  B : PMIOPort  Side=Left
  H : PMIOPort  Port=2  Side=Right
  connections:
  Base xForm/RConn1 -- B/RConn1
  Hole xForm/LConn1 -- Base xForm/LConn1 -- Bracket/LConn1
  H/RConn1 -- Hole xForm/RConn1

== system WormAndGearConstraint0x5B10x5D/Solar Array/Solar Tracker1/Drive Connection/Drive Connection ==
  Cylinder : sm_lib/Body Elements/Revolved Solid  RevolutionCrossSection=crossSection  RevolutionCrossSectionUnits=m  RevolutionExtent=Full  RevolutionAngle=180  RevolutionAngleUnits=deg  ExportConvexHullGeometry=off  InertiaType=CalculateFromGeometry  BasedOnType=Density  Density=rho  DensityUnits=kg/m^3  Mass=1  MassUnits=kg  CenterOfMass=[0 0 0]  CenterOfMassUnits=m  MomentsOfInertia=[1 1 1]  MomentsOfInertiaUnits=kg*m^2  ProductsOfInertia=[1 1 1]  ProductsOfInertiaUnits=kg*m^2  GraphicType=FromGeometry  MarkerShape=Sphere  MarkerSize=10  GraphicVisPropType=SimpleVisualProperties  GraphicDiffuseColor=color  GraphicOpacity=1.0  GraphicSpecularColor=[0.5 0.5 0.5 1.0]  GraphicAmbientColor=[0.15 0.15 0.15 1.0]  GraphicEmissiveColor=[0.0 0.0 0.0 1.0]  GraphicShininess=75  DoExposeReferenceFrame=off  SerializedFrames=<Frames><Frame><Id>Frame1</Id><Value><Name>L</Name><Origin><Source>GeometricFeature</Source><FeatureName>side surface 1</FeatureName></Origin><PrimaryAxis><DefinedDirection>+Z</DefinedDirection><Source>ReferenceFrame</Source><SourceDirection>+Z</SourceDirection><FeatureName></FeatureName></PrimaryAxis><SecondaryAxis><DefinedDirection>+X</DefinedDirection><Source>ReferenceFrame</Source><SourceDirection>+X</SourceDirection><FeatureName></FeatureName></SecondaryAxis></Value></Frame><Frame><Id>Frame2</Id><Value><Name>R</Name><Origin><Source>GeometricFeature</Source><FeatureName>side surface 3</FeatureName></Origin><PrimaryAxis><DefinedDirection>+Z</DefinedDirection><Source>ReferenceFrame</Source><SourceDirection>+Z</SourceDirection><FeatureName></FeatureName></PrimaryAxis><SecondaryAxis><DefinedDirection>+X</DefinedDirection><Source>ReferenceFrame</Source><SourceDirection>+X</SourceDirection><FeatureName></FeatureName></SecondaryAxis></Value></Frame></Frames>
  L : PMIOPort  Side=Left
  R : PMIOPort  Port=2  Side=Right
  connections:
  R/RConn1 -- Cylinder/RConn1
  Cylinder/LConn1 -- L/RConn1
